simulink model "TestSim"  (R2021a)
settings: Solver=FixedStepDiscrete  StartTime=0.0  StopTime=10.0  FixedStep=0.01  RelTol=1e-3
values from neighbouring files (symbols this model uses):
  axleLength = 0.136    [robotParameters.m]
  ticksPerRot = 20    [robotParameters.m]
  wheelR = 0.031    [robotParameters.m]
undefined symbols (not defined in the file or in its folder): DiscIntNeverNeededParam, InputPWM, lineLength, mapForSim, WheelSpeed
libraries: mobileRoboticsTrainingLib x5, pid_lib x2, simulink_extras x1
settings Model: Creator=Marc  LastModifiedBy=Marc

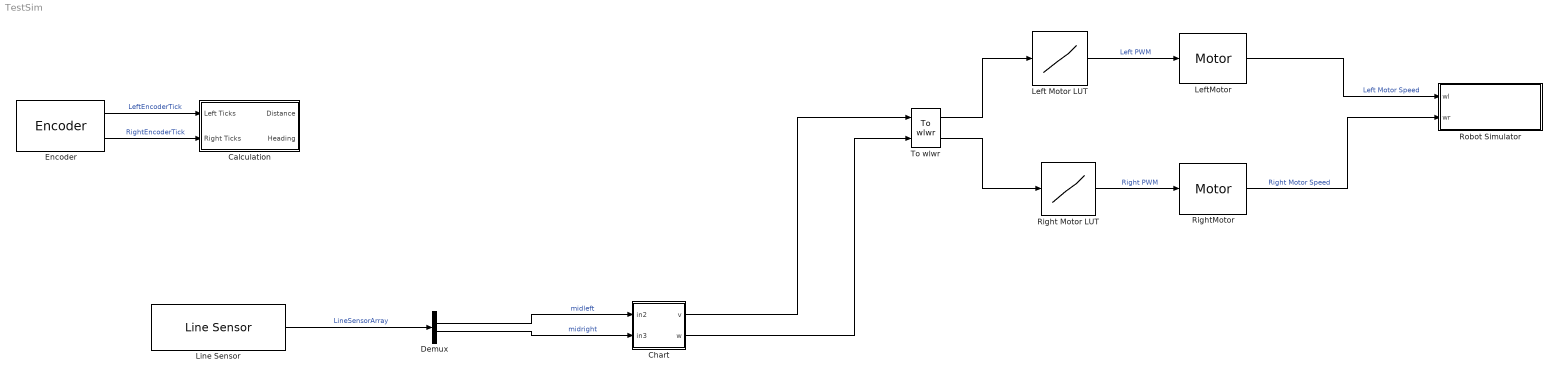
== system TestSim ==
  Calculation : Subsystem
  Chart : Stateflow chart  TreatAsAtomicUnit=on
  Demux : Demux
  Encoder : mobileRoboticsTrainingLib/Encoder  axleLength=axleLength  wheelR=wheelR  ticksPerRot=ticksPerRot
      settings: SourceProductName=Mobile Robotics Training Library
  Left Motor LUT : Lookup_n-D  NumberOfTableDimensions=1  BreakpointsForDimension1=WheelSpeed  Table=InputPWM  InterpMethod=Nearest  ExtrapMethod=Clip  InternalRulePriority=Speed  RndMeth=Simplest  InputSameDT=on
  LeftMotor : mobileRoboticsTrainingLib/Motor  motorPlant=wheelMotorModel  sensorType=Speed
      settings: SourceProductName=Mobile Robotics Training Library
  Line Sensor : mobileRoboticsTrainingLib/Line Sensor  mapVariable=mapForSim  envVal=1  lineVal=0  sensOff=[0.0643 0.0354; 0.0675 0.005; 0.0675 -0.005; 0.0643 -0.0354]
      settings: SourceProductName=Mobile Robotics Training Library
  Right Motor LUT : Lookup_n-D  NumberOfTableDimensions=1  BreakpointsForDimension1=WheelSpeed  Table=InputPWM  InterpMethod=Nearest  ExtrapMethod=Clip  InternalRulePriority=Speed  RndMeth=Simplest  InputSameDT=on
  RightMotor : mobileRoboticsTrainingLib/Motor  motorPlant=wheelMotorModel  sensorType=Speed
      settings: SourceProductName=Mobile Robotics Training Library
  Robot Simulator : Subsystem  Priority=99  AncestorBlock=mobileRoboticsTrainingLib/Robot Simulator  mask(Robot Simulator){mapVar=mapForSim, startX=0.16801, startY=0.09392, startTheta=0, axleLength=axleLength, wheelR=wheelR}
      mask prompts: mapVar "Map Variable"; startX "Start X (m)"; startY "Start Y (m)"; startTheta "Theta (deg)"; axleLength "Axle Length (m)"; wheelR "Wheel Radius (m)"
      mask help: Configure robot simulator to use custom simulation maps and simulate closed-loop mobile robotics systems along with appropriate sensor simulation blocks.
      mask init:
      | set_param(bdroot,'SolverType','Fixed-Step');
      | set_param(bdroot,'Solver','FixedStepDiscrete');
      | 
      | if (exist('Ts'))
      |     set_param(bdroot,'FixedStep','Ts');
      | else
      |     set_param(bdroot,'FixedStep','0.01');
      | end
      | 
      | h = findobj('Name','Robot Simulator');
      | if ~isempty(h)
      |     close (h);
      | end
      | setupRobotSim();
      mask Help: web('Robot Simulator.htm')
      mask DialogControl mapCont Prompt: Map Setup
      mask DialogControl initPosCont Prompt: Initial Position
      mask DialogControl setPos Prompt: Set position interactively
      mask DialogControl setPos Callback:
      | %% Set starting point
      | setStartingPoint();
      mask DialogControl initOrientation Prompt: Initial Orientation
      mask DialogControl robotCharCont Prompt: Robot Characteristics
      mask Display: disp('Robot Simulator')
  To wlwr : mobileRoboticsTrainingLib/To wlwr  axleLength=0.1  wheelR=0.05
  wires:
  Encoder/2 -> Calculation/2(Right Ticks)  "RightEncoderTick"
  Encoder/1 -> Calculation/1(Left Ticks)  "LeftEncoderTick"
  To wlwr/1 -> Left Motor LUT/1
  RightMotor/1 -> Robot Simulator/2(wr)  "Right Motor Speed"
  Left Motor LUT/1 -> LeftMotor/1  "Left PWM"
  To wlwr/2 -> Right Motor LUT/1
  Right Motor LUT/1 -> RightMotor/1  "Right PWM"
  LeftMotor/1 -> Robot Simulator/1(wl)  "Left Motor Speed"
  Line Sensor/1 -> Demux/1  "LineSensorArray"
  Demux/2 -> Chart/1(in2)  "midleft"
  Demux/3 -> Chart/2(in3)  "midright"
  Chart/1(v) -> To wlwr/1
  Chart/2(w) -> To wlwr/2

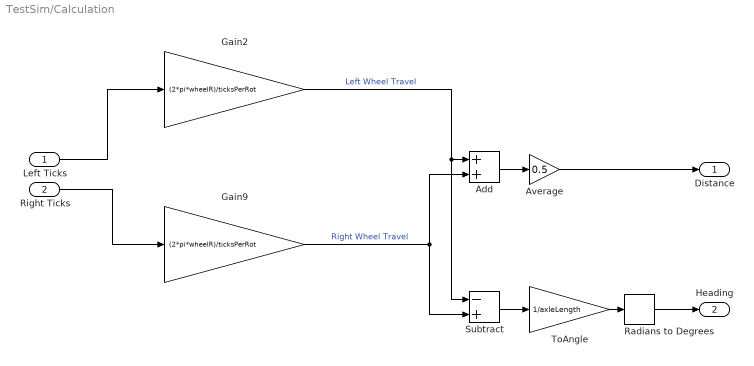
== system TestSim/Calculation ==
  Left Ticks : Inport
  Right Ticks : Inport  Port=2
  Add : Sum
  Average : Gain  Gain=0.5
  Gain2 : Gain  Gain=(2*pi*wheelR)/ticksPerRot
  Gain9 : Gain  Gain=(2*pi*wheelR)/ticksPerRot
  Radians to Degrees : simulink_extras/Transformations/Radians to Degrees
  Subtract : Sum  Inputs=-+
  ToAngle : Gain  Gain=1/axleLength
  Distance : Outport
  Heading : Outport  Port=2
  wires:
  Average/1 -> Distance/1
  Add/1 -> Average/1
  Gain2/1 -> Subtract/1, Add/1  "Left Wheel Travel"
  Right Ticks/1 -> Gain9/1
  Left Ticks/1 -> Gain2/1
  Gain9/1 -> Subtract/2, Add/2  "Right Wheel Travel"
  Subtract/1 -> ToAngle/1
  ToAngle/1 -> Radians to Degrees/1
  Radians to Degrees/1 -> Heading/1

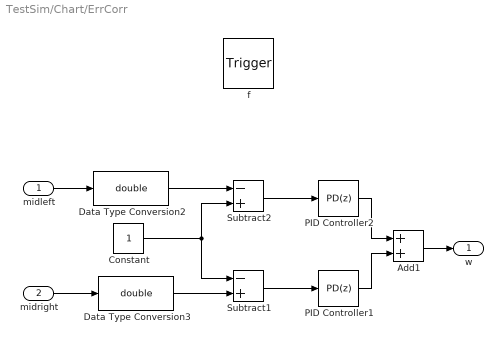
== system TestSim/Chart/ErrCorr ==
  midleft : Inport  OutDataTypeStr=double  PortDimensions=1
  midright : Inport  Port=2  OutDataTypeStr=double  PortDimensions=1
  f : TriggerPort  TriggerType=function-call  VariantControl=(inherit)
      settings: CopyFcn=Stateflow.SLINSF.SimulinkMan.removeBlockPreDeleteFcn  PreDeleteFcn=Stateflow.SLINSF.SimulinkMan.unsafePredeleteFcn
  Add1 : Sum
  Constant : Constant
  Data Type Conversion2 : DataTypeConversion  OutDataTypeStr=double
  Data Type Conversion3 : DataTypeConversion  OutDataTypeStr=double
  PID Controller1 : pid_lib/PID Controller  Controller=PD  Form=Parallel  TimeDomain=Discrete-time  UseExternalTs=off  SampleTime=-1  IntegratorMethod=Forward Euler  FilterMethod=Forward Euler  ControllerParametersSource=internal  P=1  I=1  D=1e-5  UseFilter=on  N=100  TunerSelectOption=Transfer Function Based (PID Tuner App)  InitialConditionSource=internal  InitialConditionForIntegrator=0  InitialConditionForFilter=0  DifferentiatorICPrevScaledInput=0  ExternalReset=none  TrackingMode=off  Kt=1  LimitOutput=off  SatLimitsSource=internal  UpperSaturationLimit=inf  LowerSaturationLimit=-inf  LinearizeAsGain=on  AntiWindupMode=none  Kb=1  POutMin=[]  POutMax=[]  IOutMin=[]  IOutMax=[]  DOutMin=[]  DOutMax=[]  NOutMin=[]  NOutMax=[]  SumOutMin=[]  SumOutMax=[]  SaturationOutMin=[]  SaturationOutMax=[]  PParamMin=[]  PParamMax=[]  IParamMin=[]  IParamMax=[]  DParamMin=[]  DParamMax=[]  NParamMin=[]  NParamMax=[]  KbParamMin=[]  KbParamMax=[]  KtParamMin=[]  KtParamMax=[]  KbOutMin=[]  KbOutMax=[]  KtOutMin=[]  KtOutMax=[]  IntegratorOutMin=[]  IntegratorOutMax=[]  FilterOutMin=[]  FilterOutMax=[]  SumI1OutMin=[]  SumI1OutMax=[]  SumI2OutMin=[]  SumI2OutMax=[]  SumI3OutMin=[]  SumI3OutMax=[]  SumI4OutMin=[]  SumI4OutMax=[]  SumDOutMin=[]  SumDOutMax=[]  DifferentiatorOutMin=[]  DifferentiatorOutMax=[]  FilterDiffOutCoefMin=[]  FilterDiffOutCoefMax=[]  ReciprocalOutMin=[]  ReciprocalOutMax=[]  SumDenOutMin=[]  SumDenOutMax=[]  SumNumOutMin=[]  SumNumOutMax=[]  DivideOutMin=[]  DivideOutMax=[]  UdiffTsProdOutMin=[]  UdiffTsProdOutMax=[]  NTsProdOutMin=[]  NTsProdOutMax=[]  UintegralTsProdOutMin=[]  UintegralTsProdOutMax=[]  UngainTsProdOutMin=[]  UngainTsProdOutMax=[]  IntegratorContinuousStateAttributes=''  IntegratorStateMustResolveToSignalObject=off  IntegratorRTWStateStorageClass=Auto  FilterContinuousStateAttributes=''  FilterStateMustResolveToSignalObject=off  FilterRTWStateStorageClass=Auto  ParallelPVariant=InternalParameters  IdealPVariant=Disabled  IVariant=Disabled  DVariant=InternalParameters  IntegratorVariant=Disabled  SatVariant=Disabled  AWVariant=Disabled  PCopyVariant=Disabled  TRVariant=Disabled  FdbkBlocksVariant=Forward  IdealPFdbkVariant=Disabled  SatFdbkVariant=Disabled  DerivativeFilterVariant=ForwardEulerFilter  NVariant=InternalParameters  NCopyVariant=Disabled  FilterICVariant=InternalICsFilter  IntegratorICVariant=Disabled  ExternalResetVariant=Disabled  TRSumVariant=Passthrough  SumFdbkVariant=Disabled  SumVariant=Sum_PD  TsampFilterVariant=InternalTs  TsampNgainVariant=Passthrough  TsampIntegralVariant=Disabled_SignalSpec  ExternalSaturationOutDataTypeStr=Inherit: Same as second input  InitialConditionSetting=Output
  PID Controller2 : pid_lib/PID Controller  Controller=PD  Form=Parallel  TimeDomain=Discrete-time  UseExternalTs=off  SampleTime=-1  IntegratorMethod=Forward Euler  FilterMethod=Forward Euler  ControllerParametersSource=internal  P=1  I=1  D=1e-5  UseFilter=on  N=100  TunerSelectOption=Transfer Function Based (PID Tuner App)  InitialConditionSource=internal  InitialConditionForIntegrator=0  InitialConditionForFilter=0  DifferentiatorICPrevScaledInput=0  ExternalReset=none  TrackingMode=off  Kt=1  LimitOutput=off  SatLimitsSource=internal  UpperSaturationLimit=inf  LowerSaturationLimit=-inf  LinearizeAsGain=on  AntiWindupMode=none  Kb=1  POutMin=[]  POutMax=[]  IOutMin=[]  IOutMax=[]  DOutMin=[]  DOutMax=[]  NOutMin=[]  NOutMax=[]  SumOutMin=[]  SumOutMax=[]  SaturationOutMin=[]  SaturationOutMax=[]  PParamMin=[]  PParamMax=[]  IParamMin=[]  IParamMax=[]  DParamMin=[]  DParamMax=[]  NParamMin=[]  NParamMax=[]  KbParamMin=[]  KbParamMax=[]  KtParamMin=[]  KtParamMax=[]  KbOutMin=[]  KbOutMax=[]  KtOutMin=[]  KtOutMax=[]  IntegratorOutMin=[]  IntegratorOutMax=[]  FilterOutMin=[]  FilterOutMax=[]  SumI1OutMin=[]  SumI1OutMax=[]  SumI2OutMin=[]  SumI2OutMax=[]  SumI3OutMin=[]  SumI3OutMax=[]  SumI4OutMin=[]  SumI4OutMax=[]  SumDOutMin=[]  SumDOutMax=[]  DifferentiatorOutMin=[]  DifferentiatorOutMax=[]  FilterDiffOutCoefMin=[]  FilterDiffOutCoefMax=[]  ReciprocalOutMin=[]  ReciprocalOutMax=[]  SumDenOutMin=[]  SumDenOutMax=[]  SumNumOutMin=[]  SumNumOutMax=[]  DivideOutMin=[]  DivideOutMax=[]  UdiffTsProdOutMin=[]  UdiffTsProdOutMax=[]  NTsProdOutMin=[]  NTsProdOutMax=[]  UintegralTsProdOutMin=[]  UintegralTsProdOutMax=[]  UngainTsProdOutMin=[]  UngainTsProdOutMax=[]  IntegratorContinuousStateAttributes=''  IntegratorStateMustResolveToSignalObject=off  IntegratorRTWStateStorageClass=Auto  FilterContinuousStateAttributes=''  FilterStateMustResolveToSignalObject=off  FilterRTWStateStorageClass=Auto  ParallelPVariant=InternalParameters  IdealPVariant=Disabled  IVariant=Disabled  DVariant=InternalParameters  IntegratorVariant=Disabled  SatVariant=Disabled  AWVariant=Disabled  PCopyVariant=Disabled  TRVariant=Disabled  FdbkBlocksVariant=Forward  IdealPFdbkVariant=Disabled  SatFdbkVariant=Disabled  DerivativeFilterVariant=ForwardEulerFilter  NVariant=InternalParameters  NCopyVariant=Disabled  FilterICVariant=InternalICsFilter  IntegratorICVariant=Disabled  ExternalResetVariant=Disabled  TRSumVariant=Passthrough  SumFdbkVariant=Disabled  SumVariant=Sum_PD  TsampFilterVariant=InternalTs  TsampNgainVariant=Passthrough  TsampIntegralVariant=Disabled_SignalSpec  ExternalSaturationOutDataTypeStr=Inherit: Same as second input  InitialConditionSetting=Output
  Subtract1 : Sum  Inputs=-+
  Subtract2 : Sum  Inputs=-+
  w : Outport
  wires:
  PID Controller2/1 -> Add1/1
  Subtract2/1 -> PID Controller2/1
  Subtract1/1 -> PID Controller1/1
  PID Controller1/1 -> Add1/2
  Data Type Conversion2/1 -> Subtract2/1
  Constant/1 -> Subtract2/2, Subtract1/1
  Data Type Conversion3/1 -> Subtract1/2
  Add1/1 -> w/1
  midleft/1 -> Data Type Conversion2/1
  midright/1 -> Data Type Conversion3/1

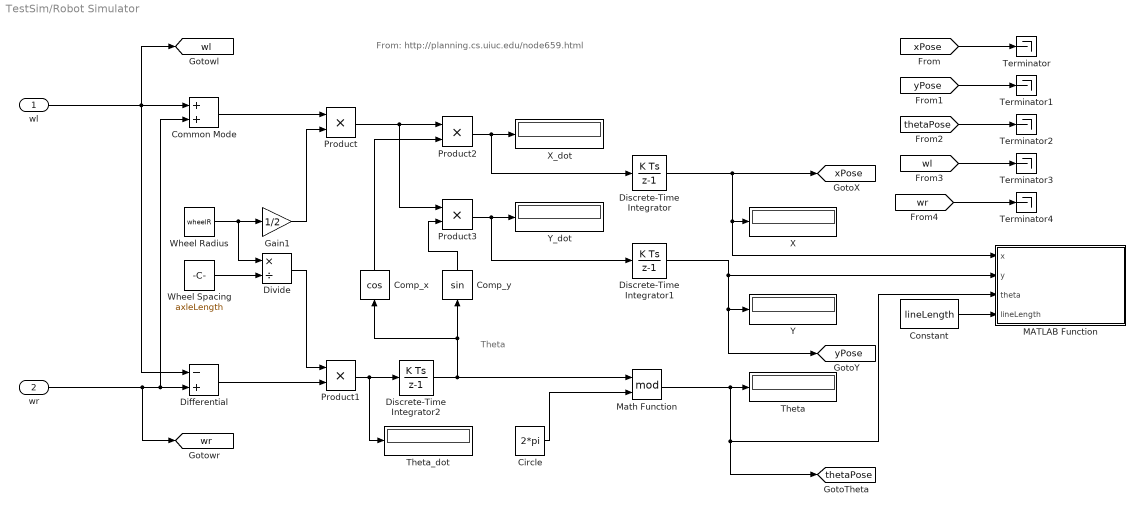
== system TestSim/Robot Simulator ==
  note: Theta
  note: From: http://planning.cs.uiuc.edu/node659.html
  wl : Inport
  wr : Inport  Port=2
  Circle : Constant  Value=2*pi
  Common Mode : Sum
  Comp_x : Trigonometry  Operator=cos
  Comp_y : Trigonometry
  Constant : Constant  Value=lineLength
  Differential : Sum  Inputs=-+
  Discrete-Time Integrator : DiscreteIntegrator  InitialCondition=startX  SampleTime=-1  ICPrevOutput=DiscIntNeverNeededParam  ICPrevScaledInput=DiscIntNeverNeededParam
  Discrete-Time Integrator1 : DiscreteIntegrator  InitialCondition=startY  SampleTime=-1  ICPrevOutput=DiscIntNeverNeededParam  ICPrevScaledInput=DiscIntNeverNeededParam
  Discrete-Time Integrator2 : DiscreteIntegrator  InitialCondition=startTheta*(pi/180)  SampleTime=-1  ICPrevOutput=DiscIntNeverNeededParam  ICPrevScaledInput=DiscIntNeverNeededParam
  Divide : Product  Inputs=*/
  Gain1 : Gain  Gain=1/2
  MATLAB Function : MATLAB Function  TreatAsAtomicUnit=on
  Math Function : Math  Operator=mod  SignedPower=on  SaturateOnIntegerOverflow=on
  Product{,1..3} (4 alike) : Product  RndMeth=Zero
  Terminator{,1..4} (5 alike) : Terminator
  Theta : Display
  Theta_dot : Display
  Wheel Radius : Constant  Value=wheelR
  Wheel Spacing : Constant  Value=axleLength
  X : Display
  X_dot : Display
  Y : Display
  Y_dot : Display
  tag scope: thetaPose=global, wl=global, wr=global, xPose=global, yPose=global
  wires:
  [wr] -> Terminator4/1
  [wl] -> Terminator3/1
  Math Function/1 -> [thetaPose], MATLAB Function/3(theta), Theta/1
  Differential/1 -> Product1/2
  Comp_y/1 -> Product3/2
  Discrete-Time Integrator/1 -> [xPose], MATLAB Function/1(x), X/1
  Product3/1 -> Discrete-Time Integrator1/1, Y_dot/1
  Discrete-Time Integrator1/1 -> Y/1, [yPose], MATLAB Function/2(y)
  Divide/1 -> Product1/1
  wr/1 -> [wr], Common Mode/2, Differential/2
  Discrete-Time Integrator2/1 -> Math Function/1, Comp_x/1, Comp_y/1
  wl/1 -> [wl], Common Mode/1, Differential/1
  Comp_x/1 -> Product2/2
  Product1/1 -> Discrete-Time Integrator2/1, Theta_dot/1
  Wheel Radius/1 -> Divide/1, Gain1/1
  Wheel Spacing/1 -> Divide/2
  Product2/1 -> Discrete-Time Integrator/1, X_dot/1
  Gain1/1 -> Product/2
  Common Mode/1 -> Product/1
  Product/1 -> Product3/1, Product2/1
  Circle/1 -> Math Function/2
  Constant/1 -> MATLAB Function/4(lineLength)
  [xPose] -> Terminator/1
  [yPose] -> Terminator1/1
  [thetaPose] -> Terminator2/1

== matlab function TestSim/Robot Simulator/MATLAB Function ==
  data: x input; y input; theta input; lineLength input
function plotRobot(x,y,theta,lineLength)
% Get plot details
coder.extrinsic('evalin','plot')
ph1 = evalin('base','PlotHandle1');
ph2 = evalin('base','PlotHandle2');

% Find length orientation line
xp = [x x+lineLength*cos(theta)];
yp = [y y+lineLength*sin(theta)];

% Plot robot
set(ph1,'xdata',xp,'ydata',yp);
set(ph2,'xdata',x,'ydata',y);
drawnow('limitrate')

== stateflow chart TestSim/Chart ==
  state w=ErrCorr(midleft,midright) [function]
  state Initial
    entry:
    v=0;
    w=0;
  state Follow
    entry,during:
    v=0.1;
    w=ErrCorr(in2,in3)
  (default) -> Initial
  Initial -> Follow : [in2==0 & in3==0]
  data: midleft function_input double size=1; midright function_input double size=1; w function_output; in2 input; in3 input; v output; w output
